simulink library "coolantFlow_lib"  (R2025a)
settings: Solver=VariableStepAuto  StartTime=0.0  StopTime=10.0  RelTol=1e-3
libraries: fl_lib x4
settings Model: Creator=mbhattu  LastModifiedBy=mbhattu

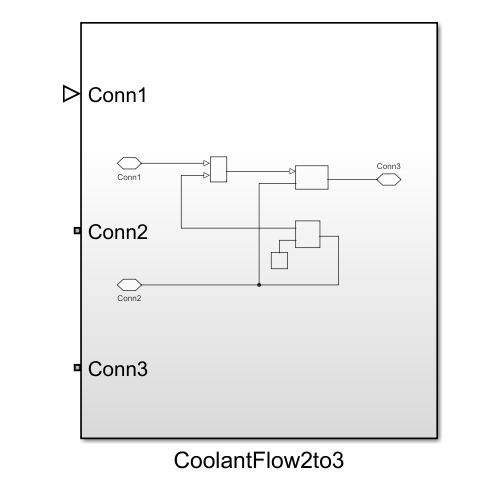
[thumbnail: Simulink's stored preview of the top-level diagram]
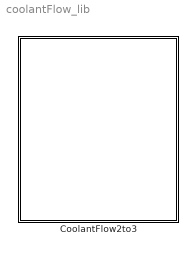
== system coolantFlow_lib ==
  CoolantFlow2to3 : Subsystem

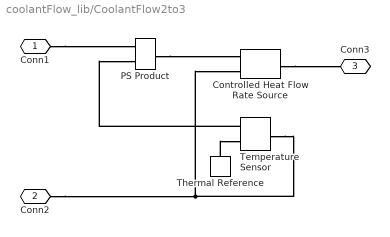
== system coolantFlow_lib/CoolantFlow2to3 ==
  Controlled Heat Flow Rate Source : fl_lib/Thermal/Thermal Sources/Controlled Heat Flow Rate Source
  PS Product : fl_lib/Physical Signals/Functions/PS Product
  Temperature Sensor : fl_lib/Thermal/Thermal Sensors/Temperature Sensor  temperature_measure=foundation.enum.MeasurementReference.difference
  Thermal Reference : fl_lib/Thermal/Thermal Elements/Thermal Reference
  Conn1 : PMIOPort  Side=Left
  Conn2 : PMIOPort  Port=2  Side=Left
  Conn3 : PMIOPort  Port=3  Side=Left
  connections:
  Temperature Sensor/RConn2 -- PS Product/LConn2
  PS Product/RConn1 -- Controlled Heat Flow Rate Source/RConn1
  Conn1/RConn1 -- PS Product/LConn1
  Temperature Sensor/LConn1 -- Conn2/RConn1 -- Controlled Heat Flow Rate Source/RConn2
  Thermal Reference/LConn1 -- Temperature Sensor/RConn1
  Controlled Heat Flow Rate Source/LConn1 -- Conn3/RConn1
